simulink subsystem "DKE_nadirpointing_magneto"  (R2021a)
settings: Solver=VariableStepAuto  StartTime=0.0  StopTime=10.0  RelTol=1e-3
undefined symbols (not defined in the file): IAU
libraries: aerolibutil x3, aerolibtransform2 x2, sharedtransform x1
settings Model: Creator=Laura  LastModifiedBy=Laura

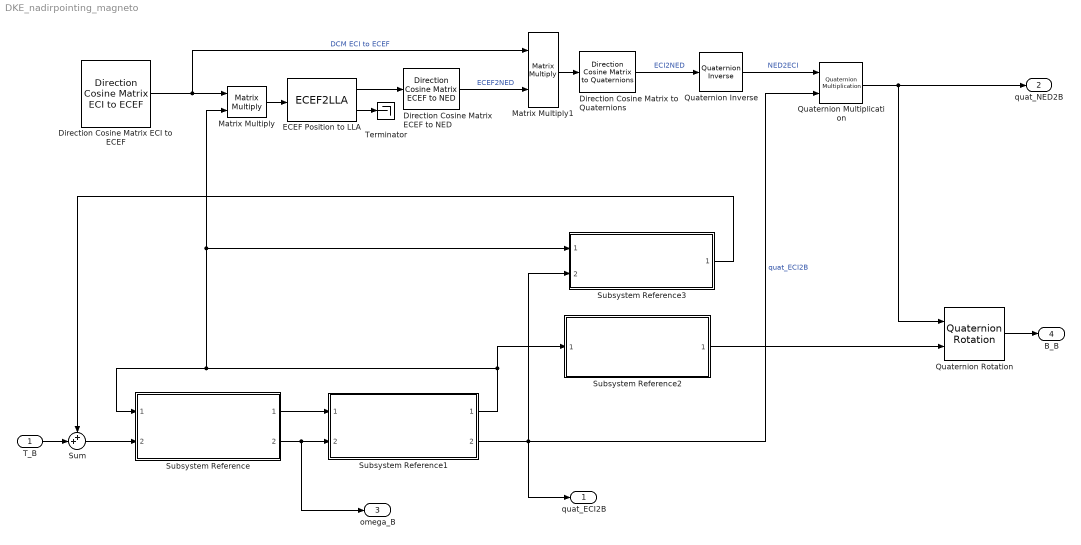
== system DKE_nadirpointing_magneto ==
  T_B : Inport
  Direction Cosine Matrix ECEF to NED : aerolibtransform2/Direction Cosine Matrix ECEF to NED
      settings: SourceProductBaseCode=AE
  Direction Cosine Matrix ECI to ECEF : aerolibtransform2/Direction Cosine Matrix ECI to ECEF  red=IAU-2000/2006  year=year  month=February  day=1  hour=hour  min=min  sec=sec  deltaT=None  errorflag=Error  extraparamflag=off
      settings: AttributesFormatString=%<red>  SourceProductBaseCode=AE
  Direction Cosine Matrix to Quaternions : sharedtransform/Direction Cosine Matrix  to Quaternions  aMode=0  action=None  tolerance=eps(2)
      settings: SourceProductBaseCode=AE,PW,DR,MT,UV,VE
  ECEF Position to LLA : ECEF2LLA
  Matrix Multiply : Product  Multiplication=Matrix(*)
  Matrix Multiply1 : Product  Multiplication=Matrix(*)
  Quaternion Inverse : aerolibutil/Quaternion Inverse
  Quaternion Multiplication : aerolibutil/Quaternion Multiplication
  Quaternion Rotation : aerolibutil/Quaternion Rotation
  Subsystem Reference : Subsystem  ReferencedSubsystem=Dynamics
  Subsystem Reference1 : Subsystem  ReferencedSubsystem=Kinematics
  Subsystem Reference2 : Subsystem  ReferencedSubsystem=MagnetoField_magneto
  Subsystem Reference3 : Subsystem  ReferencedSubsystem=GravityTorque
  Sum : Sum  Inputs=++|
  Terminator : Terminator
  quat_ECI2B : Outport
  quat_NED2B : Outport  Port=2
  omega_B : Outport  Port=3
  B_B : Outport  Port=4
  wires:
  Subsystem Reference3/1 -> Sum/1
  Quaternion Inverse/1 -> Quaternion Multiplication/1  "NED2ECI"
  Subsystem Reference/2 -> Subsystem Reference1/2, omega_B/1
  Direction Cosine Matrix to Quaternions/1 -> Quaternion Inverse/1  "ECI2NED"
  Direction Cosine Matrix ECEF to NED/1 -> Matrix Multiply1/2  "ECEF2NED"
  Quaternion Multiplication/1 -> quat_NED2B/1, Quaternion Rotation/1
  ECEF Position to LLA/1 -> Direction Cosine Matrix ECEF to NED/1
  T_B/1 -> Sum/2
  ECEF Position to LLA/2 -> Terminator/1
  Matrix Multiply/1 -> ECEF Position to LLA/1
  Subsystem Reference1/1 -> Subsystem Reference/1, Subsystem Reference3/1, Matrix Multiply/2, Subsystem Reference2/1
  Sum/1 -> Subsystem Reference/2
  Direction Cosine Matrix ECI to ECEF/1 -> Matrix Multiply/1, Matrix Multiply1/1  "DCM ECI to ECEF"
  Subsystem Reference/1 -> Subsystem Reference1/1
  Subsystem Reference1/2 -> quat_ECI2B/1, Quaternion Multiplication/2, Subsystem Reference3/2  "quat_ECI2B"
  Matrix Multiply1/1 -> Direction Cosine Matrix to Quaternions/1
  Quaternion Rotation/1 -> B_B/1
  Subsystem Reference2/1 -> Quaternion Rotation/2
